simulink model "L0204"  (R2015b)
settings: Solver=VariableStepAuto  StartTime=0.0  StopTime=10.0  RelTol=1e-3
libraries: simulink x4
settings Model: Creator=mmf.shpakAV  LastModifiedBy=mmf.shpakAV

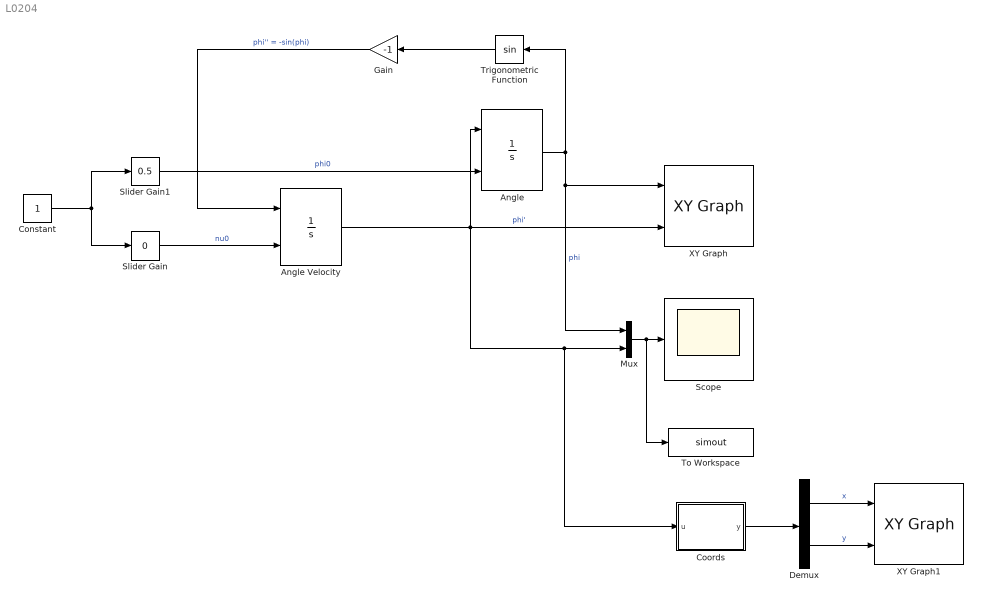
== system L0204 ==
  Angle : Integrator  InitialConditionSource=external
  Angle Velocity : Integrator  InitialConditionSource=external
  Constant : Constant
  Coords : MATLAB Function  TreatAsAtomicUnit=on
  Demux : Demux  Outputs=2
  Gain : Gain  Gain=-1
  Mux : Mux  Inputs=2
  Scope : Scope
  Slider Gain : simulink/Math Operations/Slider Gain  low=0  gain=0  high=2
  Slider Gain1 : simulink/Math Operations/Slider Gain  low=0  gain=0.5  high=2
  To Workspace : ToWorkspace  VariableName=simout  SaveFormat=Structure With Time  SampleTime=-1
  Trigonometric Function : Trigonometry
  XY Graph : simulink/Sinks/XY Graph  xmin=-1  xmax=1  ymin=-1  ymax=1  st=-1
  XY Graph1 : simulink/Sinks/XY Graph  xmin=-1  xmax=1  ymin=-1  ymax=1  st=-1
  wires:
  Angle Velocity/1 -> Angle/1, Coords/1(u), Mux/2, XY Graph/2  "phi'"
  Angle/1 -> Mux/1, XY Graph/1, Trigonometric Function/1  "phi"
  Gain/1 -> Angle Velocity/1  "phi'' = -sin(phi)"
  Mux/1 -> To Workspace/1, Scope/1
  Trigonometric Function/1 -> Gain/1
  Slider Gain/1 -> Angle Velocity/2  "nu0"
  Slider Gain1/1 -> Angle/2  "phi0"
  Demux/1 -> XY Graph1/1  "x"
  Demux/2 -> XY Graph1/2  "y"
  Coords/1(y) -> Demux/1
  Constant/1 -> Slider Gain/1, Slider Gain1/1

== matlab function L0204/Coords ==
  data: u input; y output
function y = fcn(u)
%#codegen

y = [sin(u),-cos(u)]';
